simulink model "main_model"  (R2020a)
settings: Solver=VariableStepAuto  StartTime=0.0  StopTime=25  RelTol=1e-3
model workspace (MAT data in the model file):
  Gvden1 = 1
values from neighbouring files (symbols this model uses):
  Gvnum = num(3:5)    [transfer_function.m]
undefined symbols (not defined in the file or in its folder): exp_denp, exp_nump, Gvden
libraries: simulink x11
settings Model: Creator=Ahmet  LastModifiedBy=Ahmet

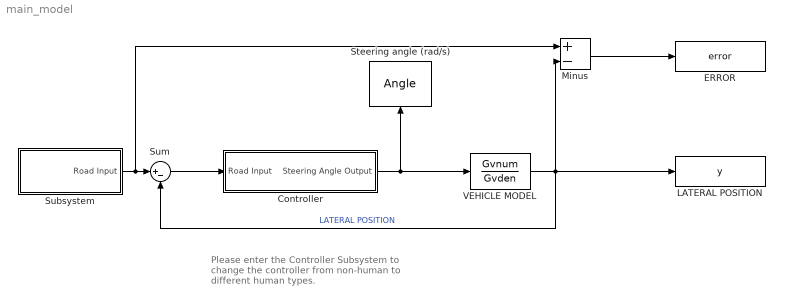
== system main_model ==
  note: Please enter the Controller Subsystem
      | to change the controller from non-human
      | to different human types.
  "Controller " : Subsystem
  ERROR : ToWorkspace  VariableName=error  SaveFormat=Timeseries  SampleTime=-1
  LATERAL POSITION : ToWorkspace  VariableName=y  SaveFormat=Timeseries  SampleTime=-1
  Minus : Sum  Inputs=+-
  Steering angle (rad/s) : ToWorkspace  VariableName=Angle  SaveFormat=Timeseries  SampleTime=-1
  Subsystem : Subsystem
  Sum : Sum  Inputs=|+-
  VEHICLE MODEL : TransferFcn  Numerator=Gvnum  Denominator=Gvden
  wires:
  VEHICLE MODEL/1 -> Sum/2, LATERAL POSITION/1, Minus/2  "LATERAL POSITION"
  Sum/1 -> "Controller "/1(Road Input)
  Subsystem/1(Road Input) -> Sum/1, Minus/1
  "Controller "/1(Steering Angle Output) -> VEHICLE MODEL/1, Steering angle (rad/s)/1
  Minus/1 -> ERROR/1

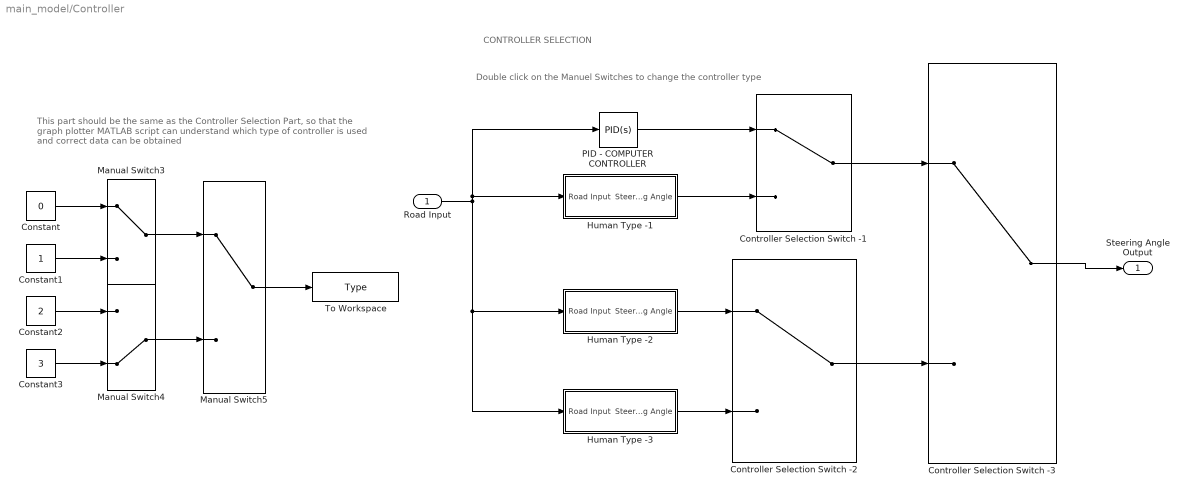
== system main_model/Controller  ==
  note: Double click on the Manuel Switches to change the controller type
  note: CONTROLLER SELECTION
  note: This part should be the same as the Controller Selection Part, so that the graph plotter MATLAB
      | script can understand which type of controller is used and correct data can be obtained
  Road Input : Inport
  Constant : Constant  Value=0
  Constant1 : Constant
  Constant2 : Constant  Value=2
  Constant3 : Constant  Value=3
  Controller Selection Switch -1 : ManualSwitch
  Controller Selection Switch -2 : ManualSwitch
  Controller Selection Switch -3 : ManualSwitch
  "Human Type -1 " : Subsystem
  Human Type -2 : Subsystem
  Human Type -3 : Subsystem
  Manual Switch3 : ManualSwitch
  Manual Switch4 : ManualSwitch  CurrentSetting=0
  Manual Switch5 : ManualSwitch
  PID - COMPUTER CONTROLLER : simulink/Continuous/PID Controller  Controller=PID  Form=Parallel  TimeDomain=Continuous-time  UseExternalTs=off  SampleTime=-1  IntegratorMethod=Forward Euler  FilterMethod=Forward Euler  ControllerParametersSource=internal  P=0.15  I=0.01  D=0.55  UseFilter=on  N=25  TunerSelectOption=Transfer Function Based (PID Tuner App)  InitialConditionSource=internal  InitialConditionForIntegrator=0  InitialConditionForFilter=0  DifferentiatorICPrevScaledInput=0  ExternalReset=none  TrackingMode=off  Kt=1  LimitOutput=off  UpperSaturationLimit=inf  LowerSaturationLimit=-inf  LinearizeAsGain=on  AntiWindupMode=none  Kb=1  POutMin=[]  POutMax=[]  IOutMin=[]  IOutMax=[]  DOutMin=[]  DOutMax=[]  NOutMin=[]  NOutMax=[]  SumOutMin=[]  SumOutMax=[]  SaturationOutMin=[]  SaturationOutMax=[]  PParamMin=[]  PParamMax=[]  IParamMin=[]  IParamMax=[]  DParamMin=[]  DParamMax=[]  NParamMin=[]  NParamMax=[]  KbParamMin=[]  KbParamMax=[]  KtParamMin=[]  KtParamMax=[]  KbOutMin=[]  KbOutMax=[]  KtOutMin=[]  KtOutMax=[]  IntegratorOutMin=[]  IntegratorOutMax=[]  FilterOutMin=[]  FilterOutMax=[]  SumI1OutMin=[]  SumI1OutMax=[]  SumI2OutMin=[]  SumI2OutMax=[]  SumI3OutMin=[]  SumI3OutMax=[]  SumI4OutMin=[]  SumI4OutMax=[]  SumDOutMin=[]  SumDOutMax=[]  DifferentiatorOutMin=[]  DifferentiatorOutMax=[]  FilterDiffOutCoefMin=[]  FilterDiffOutCoefMax=[]  ReciprocalOutMin=[]  ReciprocalOutMax=[]  SumDenOutMin=[]  SumDenOutMax=[]  SumNumOutMin=[]  SumNumOutMax=[]  DivideOutMin=[]  DivideOutMax=[]  UdiffTsProdOutMin=[]  UdiffTsProdOutMax=[]  NTsProdOutMin=[]  NTsProdOutMax=[]  UintegralTsProdOutMin=[]  UintegralTsProdOutMax=[]  UngainTsProdOutMin=[]  UngainTsProdOutMax=[]  IntegratorContinuousStateAttributes=''  IntegratorStateMustResolveToSignalObject=off  IntegratorRTWStateStorageClass=Auto  FilterContinuousStateAttributes=''  FilterStateMustResolveToSignalObject=off  FilterRTWStateStorageClass=Auto  ParallelPVariant=InternalParameters  IdealPVariant=Disabled  IVariant=InternalParameters  DVariant=InternalParameters  IntegratorVariant=Continuous  SatVariant=Disabled  AWVariant=Passthrough  PCopyVariant=Disabled  TRVariant=Disabled  FdbkBlocksVariant=Forward  IdealPFdbkVariant=Disabled  SatFdbkVariant=Disabled  DerivativeFilterVariant=ContFilter  NVariant=InternalParameters  NCopyVariant=Disabled  FilterICVariant=InternalICsFilter  IntegratorICVariant=InternalICs  ExternalResetVariant=Disabled  TRSumVariant=Passthrough  SumFdbkVariant=Disabled  SumVariant=Sum_PID  TsampFilterVariant=InternalTs  TsampNgainVariant=Passthrough  TsampIntegralVariant=Passthrough
  To Workspace : ToWorkspace  VariableName=Type  SaveFormat=Timeseries  SampleTime=-1
  Steering Angle Output : Outport
  wires:
  PID - COMPUTER CONTROLLER/1 -> Controller Selection Switch -1/1
  "Human Type -1 "/1(Steering Angle) -> Controller Selection Switch -1/2
  Road Input/1 -> PID - COMPUTER CONTROLLER/1, "Human Type -1 "/1(Road Input), Human Type -3/1(Road Input), Human Type -2/1(Road Input)
  Controller Selection Switch -1/1 -> Controller Selection Switch -3/1
  Controller Selection Switch -2/1 -> Controller Selection Switch -3/2
  Controller Selection Switch -3/1 -> Steering Angle Output/1
  Manual Switch5/1 -> To Workspace/1
  Manual Switch4/1 -> Manual Switch5/2
  Constant2/1 -> Manual Switch4/1
  Constant3/1 -> Manual Switch4/2
  Constant/1 -> Manual Switch3/1
  Constant1/1 -> Manual Switch3/2
  Manual Switch3/1 -> Manual Switch5/1
  Human Type -2/1(Steering Angle) -> Controller Selection Switch -2/1
  Human Type -3/1(Steering Angle) -> Controller Selection Switch -2/2

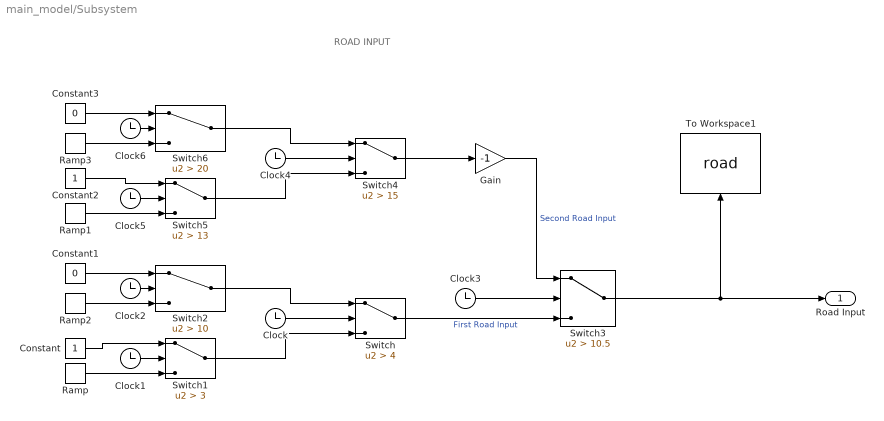
== system main_model/Subsystem ==
  note: ROAD INPUT
  Clock{,1..6} (7 alike) : Clock
  Constant : Constant
  Constant1 : Constant  Value=0
  Constant2 : Constant
  Constant3 : Constant  Value=0
  Gain : Gain  Gain=-1
  Ramp : simulink/Sources/Ramp  slope=0.5  start=1  InitialOutput=0
  Ramp1 : simulink/Sources/Ramp  slope=0.5  start=11  InitialOutput=0
  Ramp2 : simulink/Sources/Ramp  slope=-0.5  start=8  InitialOutput=1
  Ramp3 : simulink/Sources/Ramp  slope=-0.5  start=18  InitialOutput=1
  Switch : Switch  Criteria=u2 > Threshold  Threshold=4
  Switch1 : Switch  Criteria=u2 > Threshold  Threshold=3
  Switch2 : Switch  Criteria=u2 > Threshold  Threshold=10
  Switch3 : Switch  Criteria=u2 > Threshold  Threshold=10.5
  Switch4 : Switch  Criteria=u2 > Threshold  Threshold=15
  Switch5 : Switch  Criteria=u2 > Threshold  Threshold=13
  Switch6 : Switch  Criteria=u2 > Threshold  Threshold=20
  To Workspace1 : ToWorkspace  VariableName=road  SaveFormat=Timeseries  SampleTime=-1
  Road Input : Outport
  wires:
  Clock/1 -> Switch/2
  Clock2/1 -> Switch2/2
  Clock1/1 -> Switch1/2
  Switch1/1 -> Switch/3
  Switch2/1 -> Switch/1
  Ramp/1 -> Switch1/3
  Constant/1 -> Switch1/1
  Constant1/1 -> Switch2/1
  Ramp2/1 -> Switch2/3
  Switch/1 -> Switch3/3  "First Road Input"
  Switch3/1 -> To Workspace1/1, Road Input/1
  Clock3/1 -> Switch3/2
  Ramp3/1 -> Switch6/3
  Switch5/1 -> Switch4/3
  Clock6/1 -> Switch6/2
  Constant2/1 -> Switch5/1
  Ramp1/1 -> Switch5/3
  Switch6/1 -> Switch4/1
  Clock5/1 -> Switch5/2
  Constant3/1 -> Switch6/1
  Clock4/1 -> Switch4/2
  Switch4/1 -> Gain/1
  Gain/1 -> Switch3/1  "Second Road Input"

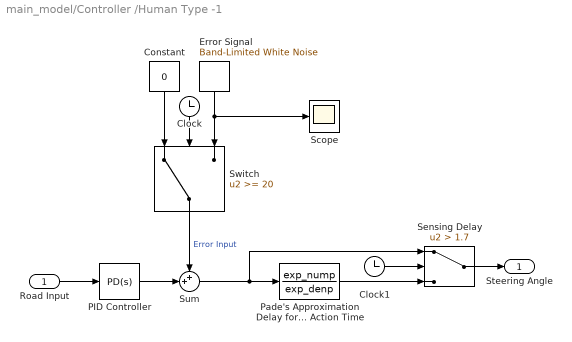
== system main_model/Controller /Human Type -1  ==
  Road Input : Inport
  Clock : Clock
  Clock1 : Clock
  Constant : Constant  Value=0
  Error Signal : simulink/Sources/Band-Limited White Noise  Cov=[0.00001]  Ts=7  seed=[23341]
  PID Controller : simulink/Continuous/PID Controller  Controller=PD  Form=Parallel  TimeDomain=Continuous-time  UseExternalTs=on  SampleTime=-1  IntegratorMethod=Forward Euler  FilterMethod=Forward Euler  ControllerParametersSource=internal  P=0.07  I=0.5  D=0.16  UseFilter=on  N=100  TunerSelectOption=Transfer Function Based (PID Tuner App)  InitialConditionSource=internal  InitialConditionForIntegrator=0  InitialConditionForFilter=0  DifferentiatorICPrevScaledInput=0  ExternalReset=none  TrackingMode=off  Kt=1  LimitOutput=off  UpperSaturationLimit=inf  LowerSaturationLimit=-inf  LinearizeAsGain=on  AntiWindupMode=none  Kb=1  POutMin=[]  POutMax=[]  IOutMin=[]  IOutMax=[]  DOutMin=[]  DOutMax=[]  NOutMin=[]  NOutMax=[]  SumOutMin=[]  SumOutMax=[]  SaturationOutMin=[]  SaturationOutMax=[]  PParamMin=[]  PParamMax=[]  IParamMin=[]  IParamMax=[]  DParamMin=[]  DParamMax=[]  NParamMin=[]  NParamMax=[]  KbParamMin=[]  KbParamMax=[]  KtParamMin=[]  KtParamMax=[]  KbOutMin=[]  KbOutMax=[]  KtOutMin=[]  KtOutMax=[]  IntegratorOutMin=[]  IntegratorOutMax=[]  FilterOutMin=[]  FilterOutMax=[]  SumI1OutMin=[]  SumI1OutMax=[]  SumI2OutMin=[]  SumI2OutMax=[]  SumI3OutMin=[]  SumI3OutMax=[]  SumI4OutMin=[]  SumI4OutMax=[]  SumDOutMin=[]  SumDOutMax=[]  DifferentiatorOutMin=[]  DifferentiatorOutMax=[]  FilterDiffOutCoefMin=[]  FilterDiffOutCoefMax=[]  ReciprocalOutMin=[]  ReciprocalOutMax=[]  SumDenOutMin=[]  SumDenOutMax=[]  SumNumOutMin=[]  SumNumOutMax=[]  DivideOutMin=[]  DivideOutMax=[]  UdiffTsProdOutMin=[]  UdiffTsProdOutMax=[]  NTsProdOutMin=[]  NTsProdOutMax=[]  UintegralTsProdOutMin=[]  UintegralTsProdOutMax=[]  UngainTsProdOutMin=[]  UngainTsProdOutMax=[]  IntegratorContinuousStateAttributes=''  IntegratorStateMustResolveToSignalObject=off  IntegratorRTWStateStorageClass=Auto  FilterContinuousStateAttributes=''  FilterStateMustResolveToSignalObject=off  FilterRTWStateStorageClass=Auto  ParallelPVariant=InternalParameters  IdealPVariant=Disabled  IVariant=Disabled  DVariant=InternalParameters  IntegratorVariant=Disabled  SatVariant=Disabled  AWVariant=Disabled  PCopyVariant=Disabled  TRVariant=Disabled  FdbkBlocksVariant=Forward  IdealPFdbkVariant=Disabled  SatFdbkVariant=Disabled  DerivativeFilterVariant=ContFilter  NVariant=InternalParameters  NCopyVariant=Disabled  FilterICVariant=InternalICsFilter  IntegratorICVariant=Disabled  ExternalResetVariant=Disabled  TRSumVariant=Passthrough  SumFdbkVariant=Disabled  SumVariant=Sum_PD  TsampFilterVariant=InternalTs  TsampNgainVariant=Passthrough  TsampIntegralVariant=Disabled_SignalSpec
  Pade's Approximation Delay for Action Time : TransferFcn  Numerator=exp_nump  Denominator=exp_denp
  Scope : Scope
  "Sensing Delay " : Switch  Criteria=u2 > Threshold  Threshold=1.7
  Sum : Sum  Inputs=++|
  Switch : Switch  Threshold=20
  Steering Angle : Outport
  wires:
  Road Input/1 -> PID Controller/1
  PID Controller/1 -> Sum/2
  Switch/1 -> Sum/1  "Error Input"
  Error Signal/1 -> Scope/1, Switch/3
  Constant/1 -> Switch/1
  Clock/1 -> Switch/2
  Sum/1 -> Pade's Approximation Delay for Action Time/1, "Sensing Delay "/1
  Pade's Approximation Delay for Action Time/1 -> "Sensing Delay "/3
  "Sensing Delay "/1 -> Steering Angle/1
  Clock1/1 -> "Sensing Delay "/2

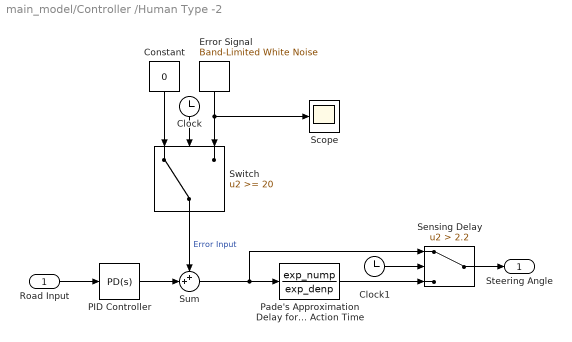
== system main_model/Controller /Human Type -2 ==
  Road Input : Inport
  Clock : Clock
  Clock1 : Clock
  Constant : Constant  Value=0
  Error Signal : simulink/Sources/Band-Limited White Noise  Cov=[0.00001]  Ts=7  seed=[23341]
  PID Controller : simulink/Continuous/PID Controller  Controller=PD  Form=Parallel  TimeDomain=Continuous-time  UseExternalTs=on  SampleTime=-1  IntegratorMethod=Forward Euler  FilterMethod=Forward Euler  ControllerParametersSource=internal  P=0.07  I=0.5  D=0.16  UseFilter=on  N=100  TunerSelectOption=Transfer Function Based (PID Tuner App)  InitialConditionSource=internal  InitialConditionForIntegrator=0  InitialConditionForFilter=0  DifferentiatorICPrevScaledInput=0  ExternalReset=none  TrackingMode=off  Kt=1  LimitOutput=off  UpperSaturationLimit=inf  LowerSaturationLimit=-inf  LinearizeAsGain=on  AntiWindupMode=none  Kb=1  POutMin=[]  POutMax=[]  IOutMin=[]  IOutMax=[]  DOutMin=[]  DOutMax=[]  NOutMin=[]  NOutMax=[]  SumOutMin=[]  SumOutMax=[]  SaturationOutMin=[]  SaturationOutMax=[]  PParamMin=[]  PParamMax=[]  IParamMin=[]  IParamMax=[]  DParamMin=[]  DParamMax=[]  NParamMin=[]  NParamMax=[]  KbParamMin=[]  KbParamMax=[]  KtParamMin=[]  KtParamMax=[]  KbOutMin=[]  KbOutMax=[]  KtOutMin=[]  KtOutMax=[]  IntegratorOutMin=[]  IntegratorOutMax=[]  FilterOutMin=[]  FilterOutMax=[]  SumI1OutMin=[]  SumI1OutMax=[]  SumI2OutMin=[]  SumI2OutMax=[]  SumI3OutMin=[]  SumI3OutMax=[]  SumI4OutMin=[]  SumI4OutMax=[]  SumDOutMin=[]  SumDOutMax=[]  DifferentiatorOutMin=[]  DifferentiatorOutMax=[]  FilterDiffOutCoefMin=[]  FilterDiffOutCoefMax=[]  ReciprocalOutMin=[]  ReciprocalOutMax=[]  SumDenOutMin=[]  SumDenOutMax=[]  SumNumOutMin=[]  SumNumOutMax=[]  DivideOutMin=[]  DivideOutMax=[]  UdiffTsProdOutMin=[]  UdiffTsProdOutMax=[]  NTsProdOutMin=[]  NTsProdOutMax=[]  UintegralTsProdOutMin=[]  UintegralTsProdOutMax=[]  UngainTsProdOutMin=[]  UngainTsProdOutMax=[]  IntegratorContinuousStateAttributes=''  IntegratorStateMustResolveToSignalObject=off  IntegratorRTWStateStorageClass=Auto  FilterContinuousStateAttributes=''  FilterStateMustResolveToSignalObject=off  FilterRTWStateStorageClass=Auto  ParallelPVariant=InternalParameters  IdealPVariant=Disabled  IVariant=Disabled  DVariant=InternalParameters  IntegratorVariant=Disabled  SatVariant=Disabled  AWVariant=Disabled  PCopyVariant=Disabled  TRVariant=Disabled  FdbkBlocksVariant=Forward  IdealPFdbkVariant=Disabled  SatFdbkVariant=Disabled  DerivativeFilterVariant=ContFilter  NVariant=InternalParameters  NCopyVariant=Disabled  FilterICVariant=InternalICsFilter  IntegratorICVariant=Disabled  ExternalResetVariant=Disabled  TRSumVariant=Passthrough  SumFdbkVariant=Disabled  SumVariant=Sum_PD  TsampFilterVariant=InternalTs  TsampNgainVariant=Passthrough  TsampIntegralVariant=Disabled_SignalSpec
  Pade's Approximation Delay for Action Time : TransferFcn  Numerator=exp_nump  Denominator=exp_denp
  Scope : Scope
  "Sensing Delay " : Switch  Criteria=u2 > Threshold  Threshold=2.2
  Sum : Sum  Inputs=++|
  Switch : Switch  Threshold=20
  Steering Angle : Outport
  wires:
  Road Input/1 -> PID Controller/1
  PID Controller/1 -> Sum/2
  Switch/1 -> Sum/1  "Error Input"
  Error Signal/1 -> Scope/1, Switch/3
  Constant/1 -> Switch/1
  Clock/1 -> Switch/2
  Sum/1 -> Pade's Approximation Delay for Action Time/1, "Sensing Delay "/1
  Pade's Approximation Delay for Action Time/1 -> "Sensing Delay "/3
  "Sensing Delay "/1 -> Steering Angle/1
  Clock1/1 -> "Sensing Delay "/2

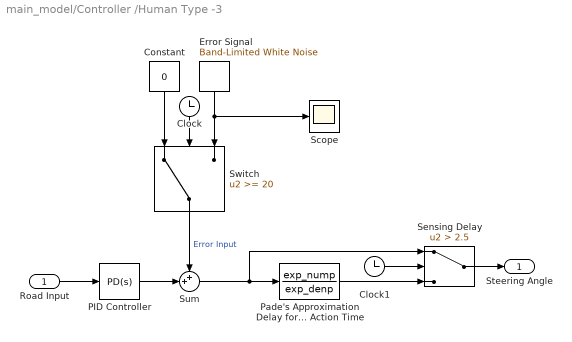
== system main_model/Controller /Human Type -3 ==
  Road Input : Inport
  Clock : Clock
  Clock1 : Clock
  Constant : Constant  Value=0
  Error Signal : simulink/Sources/Band-Limited White Noise  Cov=[0.00001]  Ts=7  seed=[23341]
  PID Controller : simulink/Continuous/PID Controller  Controller=PD  Form=Parallel  TimeDomain=Continuous-time  UseExternalTs=on  SampleTime=-1  IntegratorMethod=Forward Euler  FilterMethod=Forward Euler  ControllerParametersSource=internal  P=0.07  I=0.5  D=0.16  UseFilter=on  N=100  TunerSelectOption=Transfer Function Based (PID Tuner App)  InitialConditionSource=internal  InitialConditionForIntegrator=0  InitialConditionForFilter=0  DifferentiatorICPrevScaledInput=0  ExternalReset=none  TrackingMode=off  Kt=1  LimitOutput=off  UpperSaturationLimit=inf  LowerSaturationLimit=-inf  LinearizeAsGain=on  AntiWindupMode=none  Kb=1  POutMin=[]  POutMax=[]  IOutMin=[]  IOutMax=[]  DOutMin=[]  DOutMax=[]  NOutMin=[]  NOutMax=[]  SumOutMin=[]  SumOutMax=[]  SaturationOutMin=[]  SaturationOutMax=[]  PParamMin=[]  PParamMax=[]  IParamMin=[]  IParamMax=[]  DParamMin=[]  DParamMax=[]  NParamMin=[]  NParamMax=[]  KbParamMin=[]  KbParamMax=[]  KtParamMin=[]  KtParamMax=[]  KbOutMin=[]  KbOutMax=[]  KtOutMin=[]  KtOutMax=[]  IntegratorOutMin=[]  IntegratorOutMax=[]  FilterOutMin=[]  FilterOutMax=[]  SumI1OutMin=[]  SumI1OutMax=[]  SumI2OutMin=[]  SumI2OutMax=[]  SumI3OutMin=[]  SumI3OutMax=[]  SumI4OutMin=[]  SumI4OutMax=[]  SumDOutMin=[]  SumDOutMax=[]  DifferentiatorOutMin=[]  DifferentiatorOutMax=[]  FilterDiffOutCoefMin=[]  FilterDiffOutCoefMax=[]  ReciprocalOutMin=[]  ReciprocalOutMax=[]  SumDenOutMin=[]  SumDenOutMax=[]  SumNumOutMin=[]  SumNumOutMax=[]  DivideOutMin=[]  DivideOutMax=[]  UdiffTsProdOutMin=[]  UdiffTsProdOutMax=[]  NTsProdOutMin=[]  NTsProdOutMax=[]  UintegralTsProdOutMin=[]  UintegralTsProdOutMax=[]  UngainTsProdOutMin=[]  UngainTsProdOutMax=[]  IntegratorContinuousStateAttributes=''  IntegratorStateMustResolveToSignalObject=off  IntegratorRTWStateStorageClass=Auto  FilterContinuousStateAttributes=''  FilterStateMustResolveToSignalObject=off  FilterRTWStateStorageClass=Auto  ParallelPVariant=InternalParameters  IdealPVariant=Disabled  IVariant=Disabled  DVariant=InternalParameters  IntegratorVariant=Disabled  SatVariant=Disabled  AWVariant=Disabled  PCopyVariant=Disabled  TRVariant=Disabled  FdbkBlocksVariant=Forward  IdealPFdbkVariant=Disabled  SatFdbkVariant=Disabled  DerivativeFilterVariant=ContFilter  NVariant=InternalParameters  NCopyVariant=Disabled  FilterICVariant=InternalICsFilter  IntegratorICVariant=Disabled  ExternalResetVariant=Disabled  TRSumVariant=Passthrough  SumFdbkVariant=Disabled  SumVariant=Sum_PD  TsampFilterVariant=InternalTs  TsampNgainVariant=Passthrough  TsampIntegralVariant=Disabled_SignalSpec
  Pade's Approximation Delay for Action Time : TransferFcn  Numerator=exp_nump  Denominator=exp_denp
  Scope : Scope
  "Sensing Delay " : Switch  Criteria=u2 > Threshold  Threshold=2.5
  Sum : Sum  Inputs=++|
  Switch : Switch  Threshold=20
  Steering Angle : Outport
  wires:
  Road Input/1 -> PID Controller/1
  PID Controller/1 -> Sum/2
  Switch/1 -> Sum/1  "Error Input"
  Error Signal/1 -> Scope/1, Switch/3
  Constant/1 -> Switch/1
  Clock/1 -> Switch/2
  Sum/1 -> Pade's Approximation Delay for Action Time/1, "Sensing Delay "/1
  Pade's Approximation Delay for Action Time/1 -> "Sensing Delay "/3
  "Sensing Delay "/1 -> Steering Angle/1
  Clock1/1 -> "Sensing Delay "/2
